simulink model "Lab1"  (R2022a)
settings: Solver=VariableStepAuto  StartTime=0.0  StopTime=10  RelTol=1e-3
values from neighbouring files (symbols this model uses):
  A = 133.3    [variables.m]
  B = 0.7094    [variables.m]
  C = 0.491    [variables.m]
  eff = 1    [variables.m]
  mi = mc*(0.04 + 0.0025*ng^2)    (= 306.75849925)    [variables.m]
  ng = 8.19    [variables.m]
  r = 0.315    [variables.m]
settings Model: Creator=auamai  LastModifiedBy=auamai

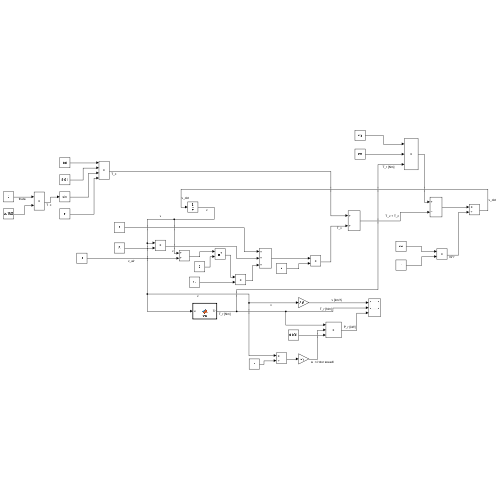
[thumbnail: Simulink's stored preview of the top-level diagram]
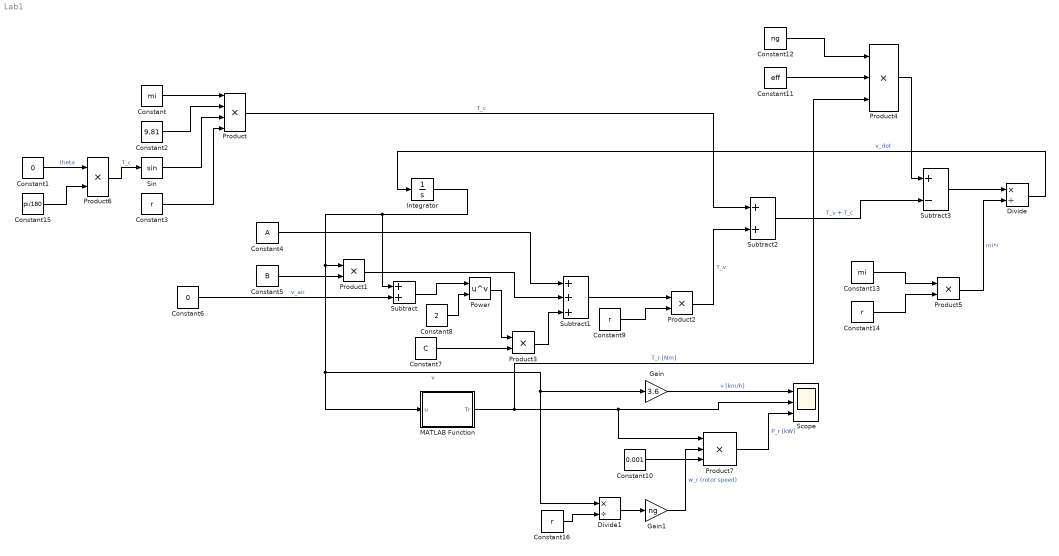
== system Lab1 ==
  Constant : Constant  Value=mi
  Constant1 : Constant  Value=0
  Constant10 : Constant  Value=0.001
  Constant11 : Constant  Value=eff
  Constant12 : Constant  Value=ng
  Constant13 : Constant  Value=mi
  Constant{3,9,14,16} (4 alike) : Constant  Value=r
  Constant15 : Constant  Value=pi/180
  Constant2 : Constant  Value=9.81
  Constant4 : Constant  Value=A
  Constant5 : Constant  Value=B
  Constant6 : Constant  Value=0
  Constant7 : Constant  Value=C
  Constant8 : Constant  Value=2
  Divide : Product  Inputs=*/
  Divide1 : Product  Inputs=*/
  Gain : Gain  Gain=3.6
  Gain1 : Gain  Gain=ng
  Integrator : Integrator
  MATLAB Function : MATLAB Function  TreatAsAtomicUnit=on
  Power : Math  Operator=pow
  Product : Product  Inputs=4
  Product{1..3,5..6} (5 alike) : Product
  Product4 : Product  Inputs=3
  Product7 : Product  Inputs=3
  Scope : Scope  NumInputPorts=3
  Sin : Trigonometry
  Subtract : Sum
  Subtract1 : Sum  Inputs=+++
  Subtract2 : Sum
  Subtract3 : Sum  Inputs=+-
  wires:
  Constant1/1 -> Product6/1  "theta"
  Constant/1 -> Product/1
  Constant2/1 -> Product/2
  Sin/1 -> Product/3
  Product/1 -> Subtract2/1  "T_c"
  Constant3/1 -> Product/4
  Divide/1 -> Integrator/1  "v_dot"
  Integrator/1 -> Subtract/1, Divide1/1, Gain/1, MATLAB Function/1(u), Product1/1  "v"
  Constant6/1 -> Subtract/2  "v_air"
  Constant5/1 -> Product1/2
  Subtract/1 -> Power/1
  Constant8/1 -> Power/2
  Constant4/1 -> Subtract1/1
  Product1/1 -> Subtract1/2
  Power/1 -> Product3/1
  Constant7/1 -> Product3/2
  Product3/1 -> Subtract1/3
  Subtract1/1 -> Product2/1
  Constant9/1 -> Product2/2
  Product2/1 -> Subtract2/2  "T_v"
  Subtract2/1 -> Subtract3/2  "T_v + T_c"
  Constant12/1 -> Product4/1
  Constant11/1 -> Product4/2
  Product4/1 -> Subtract3/1
  Subtract3/1 -> Divide/1
  Constant13/1 -> Product5/1
  Constant14/1 -> Product5/2
  Product5/1 -> Divide/2  "mi*r"
  MATLAB Function/1(Tr) -> Product4/3, Product7/1, Scope/2  "T_r [Nm]"
  Constant15/1 -> Product6/2
  Product6/1 -> Sin/1  "T_c"
  Constant16/1 -> Divide1/2
  Divide1/1 -> Gain1/1
  Product7/1 -> Scope/3  "P_r [kW]"
  Gain/1 -> Scope/1  "v [km/h]"
  Gain1/1 -> Product7/2  "w_r (rotor speed)"
  Constant10/1 -> Product7/3

== matlab function Lab1/MATLAB Function ==
  data: u input; Tr output
function Tr = fcn(u)

if u < 12.1139
    Tr = 254;
elseif u <= 40
    Tr = 80000/((u/0.315)*8.19);%80000 divided by angular velocity of the rotor
    %angular velocity of the rotor is angular velocity of the wheel times
    %the number of gears 
else
    Tr = 0;
end
